simulink model "unicycle_sd_mpc"  (R2021b)
settings: Solver=FixedStepAuto  StartTime=0.0  StopTime=simTime  RelTol=1e-3
values from neighbouring files (symbols this model uses):
  delta = Ts    [ChainedForm_mr.m]    (also in ChainedForm_sr.m = 1; initMoh.m = 1)
  deltabar = delta/2    (= 0.5)    [initMoh.m]
  ref0 = [0 0]    [initMoh.m]
  thetareference = pi/4    (= 0.785398163397)    [initMoh.m]
  Ts = deltabar    (= 0.5)    [initMoh.m]
  v0 = 0.5    [initMoh.m]
  x0 = [x01;x02;x03]    [initMoh.m]
libraries: mpclib x3
settings Model: Creator=mebbaid  LastModifiedBy=mebbaid
settings SolverCC: AlgebraicLoopSolver=TrustRegion
settings DataIOCC: ReturnWorkspaceOutputs=off
settings DebuggingCC: SignalInfNanChecking=error  SignalRangeChecking=error  ParameterUnderflowMsg=error  UniqueDataStoreMsg=error  SFMachineParentedDataDiag=warning  UnderSpecifiedDimensionMsg=warning  ArithmeticOperatorsInVariantConditions=warning
settings SFSimCC: CustomCodeUndefinedFunction=UseInterfaceOnly

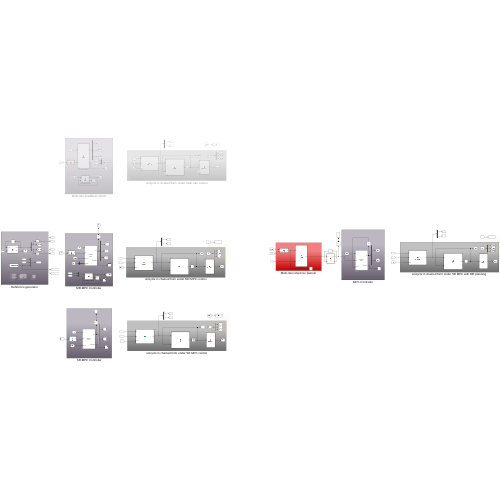
[thumbnail: Simulink's stored preview of the top-level diagram]
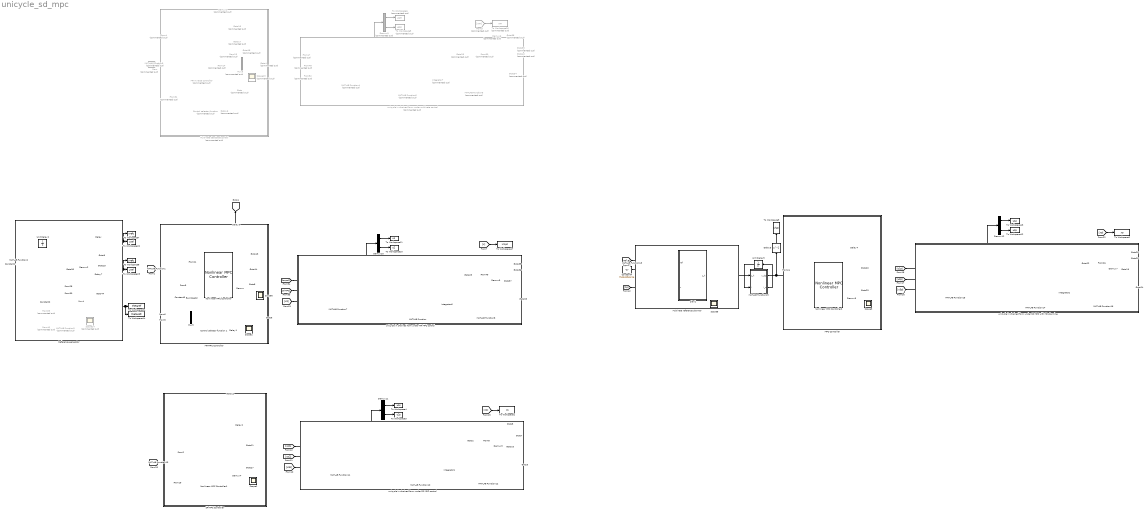
== system unicycle_sd_mpc ==
  Bus Creator : BusCreator  Inputs=1  OutDataTypeStr=Bus: myBusObject  NonVirtualBus=on
      settings: InheritFromInputs=off
  Constant1 : Constant  Value=v0
  Constant2 : Constant  Value=thetareference
  Constant3 : Constant  Value=Ts
  Constant4 : Constant  Value=thetareference
  "Control selector function " : MATLAB Function  Commented=on  TreatAsAtomicUnit=on  SystemSampleTime=deltabar
  Control selector function 1 : MATLAB Function  TreatAsAtomicUnit=on  SystemSampleTime=deltabar
  Delay : Delay  DelayLength=1  SampleTime=deltabar
  Delay1 : Delay  DelayLength=1  InitialCondition=1  SampleTime=deltabar
  Delay2 : Delay  DelayLength=1  InitialCondition=[0;0]  SampleTime=deltabar
  Delay3 : Delay  DelayLength=1  InitialCondition=[0;0;0]  SampleTime=delta
  Delay4 : Delay  DelayLength=1  InitialCondition=[0;0]  SampleTime=deltabar
  Delay5 : Delay  DelayLength=1  InitialCondition=[0 0 0]  SampleTime=delta
  Delay6 : Delay  Commented=on  DelayLength=1  InitialCondition=1  SampleTime=deltabar
  Delay7 : Delay  DelayLength=1  SampleTime=deltabar
  Demux{,3,5,7} (4 alike) : Demux  Outputs=3
  Demux1 : Demux  Commented=on  Outputs=3
  Demux{2,4,8,10..12} (6 alike) : Demux  Outputs=2
  Demux6 : Demux  Commented=on  Outputs=3
  Demux9 : Demux  Commented=on  Outputs=2
  From : From  Commented=on  GotoTag=refdes
  From13 : From  Commented=on  GotoTag=u21
  From14 : From  Commented=on  GotoTag=u22
  From3 : From  Commented=on  GotoTag=xm
  From31 : From  Commented=on  GotoTag=u2m
  From39 : From  Commented=on  GotoTag=xd
  From4 : From  Commented=on  GotoTag=zm
  From40 : From  Commented=on  GotoTag=yd
  From47 : From  Commented=on  GotoTag=u1
  From48 : From  Commented=on  GotoTag=u2_m
  From50 : From  Commented=on  GotoTag=xm
  From52 : From  Commented=on  GotoTag=x33
  Goto : Goto  Commented=on  GotoTag=u2_m
  Goto16 : Goto  Commented=on  GotoTag=u1
  Goto17 : Goto  Commented=on  GotoTag=u21
  Goto18 : Goto  Commented=on  GotoTag=u22
  Goto26 : Goto  Commented=on  GotoTag=xm
  Goto34 : Goto  Commented=on  GotoTag=zm
  Goto38 : Goto  Commented=on  GotoTag=x11
  Goto39 : Goto  Commented=on  GotoTag=x22
  Goto4 : Goto  Commented=on  GotoTag=u2m
  Goto40 : Goto  Commented=on  GotoTag=x33
  Integrator1 : Integrator  InitialCondition=x0
  Integrator2 : Integrator  InitialCondition=x0
  Integrator6 : Integrator  InitialCondition=x0
  Integrator7 : Integrator  Commented=on  InitialCondition=x0
  MATLAB Function : MATLAB Function  TreatAsAtomicUnit=on
  MATLAB Function1 : MATLAB Function  TreatAsAtomicUnit=on
  MATLAB Function10 : MATLAB Function  TreatAsAtomicUnit=on
  MATLAB Function11 : MATLAB Function  TreatAsAtomicUnit=on
  MATLAB Function12 : MATLAB Function  TreatAsAtomicUnit=on
  MATLAB Function13 : MATLAB Function  TreatAsAtomicUnit=on  SystemSampleTime=delta
  MATLAB Function14 : MATLAB Function  TreatAsAtomicUnit=on
  MATLAB Function15 : MATLAB Function  TreatAsAtomicUnit=on
  MATLAB Function16 : MATLAB Function  TreatAsAtomicUnit=on
  MATLAB Function18 : MATLAB Function  TreatAsAtomicUnit=on
  MATLAB Function19 : MATLAB Function  TreatAsAtomicUnit=on  SystemSampleTime=deltabar
  MATLAB Function2 : MATLAB Function  TreatAsAtomicUnit=on  SystemSampleTime=delta
  MATLAB Function3 : MATLAB Function  Commented=on  TreatAsAtomicUnit=on
  MATLAB Function4 : MATLAB Function  Commented=on  TreatAsAtomicUnit=on
  MATLAB Function5 : MATLAB Function  Commented=on  TreatAsAtomicUnit=on
  MATLAB Function6 : MATLAB Function  Commented=on  TreatAsAtomicUnit=on
  MATLAB Function7 : MATLAB Function  TreatAsAtomicUnit=on
  MATLAB Function8 : MATLAB Function  TreatAsAtomicUnit=on
  MATLAB Function9 : MATLAB Function  Commented=on  TreatAsAtomicUnit=on
  MPC Controller : Subsystem
  MR Inverse controller : MATLAB Function  Commented=on  TreatAsAtomicUnit=on  SystemSampleTime=delta
  MR-MPC Controller : Subsystem
  Multi-rate deadbeat control : Subsystem  Commented=on
  Multi-rate reference planner : Subsystem
  Mux3 : Mux  Commented=on  Inputs=2
  Mux4 : Mux  Inputs=3
  Mux5 : Mux  Inputs=2
  Nonlinear MPC Controller : mpclib/Nonlinear MPC Controller  SCDEnableBlockLinearizationSpecification=on  nlmpcobj=nlobj  UseObjectTs=on  TsControl=deltabar  UseMEX=off  md_enabled=off  mvtarget_enabled=off  param_enabled=on  cost_enabled=off  mvseq_enabled=off  stateseq_enabled=off  ovseq_enabled=off  slack_enabled=off  status_enabled=on  ov_min=off  ov_max=off  mv_min=off  mv_max=off  mvrate_min=off  mvrate_max=off  state_min=off  state_max=off  ov_weight=off  mv_weight=off  mvrate_weight=off  ecr_weight=off  nlp_initialize=off
  Nonlinear MPC Controller1 : mpclib/Nonlinear MPC Controller  SCDEnableBlockLinearizationSpecification=on  nlmpcobj=nlobjs  UseObjectTs=off  TsControl=deltabar  UseMEX=off  md_enabled=off  mvtarget_enabled=off  param_enabled=off  cost_enabled=off  mvseq_enabled=off  stateseq_enabled=off  ovseq_enabled=off  slack_enabled=off  status_enabled=on  ov_min=off  ov_max=off  mv_min=off  mv_max=off  mvrate_min=off  mvrate_max=off  state_min=off  state_max=off  ov_weight=off  mv_weight=off  mvrate_weight=off  ecr_weight=off  nlp_initialize=off
  Nonlinear MPC Controller2 : mpclib/Nonlinear MPC Controller  SCDEnableBlockLinearizationSpecification=on  nlmpcobj=nlobjp  UseObjectTs=on  TsControl=deltabar  UseMEX=off  md_enabled=off  mvtarget_enabled=off  param_enabled=off  cost_enabled=off  mvseq_enabled=off  stateseq_enabled=off  ovseq_enabled=off  slack_enabled=off  status_enabled=on  ov_min=off  ov_max=off  mv_min=off  mv_max=off  mvrate_min=off  mvrate_max=off  state_min=off  state_max=off  ov_weight=off  mv_weight=off  mvrate_weight=off  ecr_weight=off  nlp_initialize=off
  Reference generator : Subsystem
  SR-MPC Controller : Subsystem
  Scope{1..3,5..6} (5 alike) : Scope
  Scope13 : Scope  Commented=on
  Scope14 : Scope  Commented=on
  To Workspace1 : ToWorkspace  VariableName=xs  SampleTime=10^-3
      settings: Save2DSignal=2-D array (concatenate along first dimension)
  To Workspace10 : ToWorkspace  VariableName=u2  SampleTime=10^-3
      settings: Save2DSignal=2-D array (concatenate along first dimension)
  To Workspace11 : ToWorkspace  VariableName=u1  SampleTime=10^-3
      settings: Save2DSignal=2-D array (concatenate along first dimension)
  To Workspace12 : ToWorkspace  VariableName=u2p  SampleTime=10^-3
      settings: Save2DSignal=2-D array (concatenate along first dimension)
  To Workspace13 : ToWorkspace  VariableName=u1p  SampleTime=10^-3
      settings: Save2DSignal=2-D array (concatenate along first dimension)
  To Workspace14 : ToWorkspace  VariableName=thetarefc  SampleTime=10^-3
      settings: Save2DSignal=2-D array (concatenate along first dimension)
  To Workspace16 : ToWorkspace  Commented=on  VariableName=xm  SampleTime=10^-3
      settings: Save2DSignal=2-D array (concatenate along first dimension)
  To Workspace17 : ToWorkspace  VariableName=xmpc  SampleTime=10^-3
      settings: Save2DSignal=2-D array (concatenate along first dimension)
  To Workspace2 : ToWorkspace  VariableName=xp  SampleTime=10^-3
      settings: Save2DSignal=2-D array (concatenate along first dimension)
  To Workspace22 : ToWorkspace  VariableName=xref  SampleTime=delta
      settings: Save2DSignal=2-D array (concatenate along first dimension)
  To Workspace23 : ToWorkspace  VariableName=yref  SampleTime=delta
      settings: Save2DSignal=2-D array (concatenate along first dimension)
  To Workspace24 : ToWorkspace  VariableName=thetaref  SampleTime=delta
      settings: Save2DSignal=2-D array (concatenate along first dimension)
  To Workspace3 : ToWorkspace  VariableName=u2s  SampleTime=10^-3
      settings: Save2DSignal=2-D array (concatenate along first dimension)
  To Workspace4 : ToWorkspace  VariableName=u1s  SampleTime=10^-3
      settings: Save2DSignal=2-D array (concatenate along first dimension)
  To Workspace5 : ToWorkspace  Commented=on  VariableName=u2m  SampleTime=10^-3
      settings: Save2DSignal=2-D array (concatenate along first dimension)
  To Workspace6 : ToWorkspace  Commented=on  VariableName=u1m  SampleTime=10^-3
      settings: Save2DSignal=2-D array (concatenate along first dimension)
  To Workspace7 : ToWorkspace  VariableName=xrefc  SampleTime=10^-3
      settings: Save2DSignal=2-D array (concatenate along first dimension)
  To Workspace8 : ToWorkspace  VariableName=yrefc  SampleTime=10^-3
      settings: Save2DSignal=2-D array (concatenate along first dimension)
  To Workspace9 : ToWorkspace  VariableName=yhat  SampleTime=delta
      settings: Save2DSignal=2-D array (concatenate along first dimension)
  Unit Delay2 : UnitDelay  InitialCondition=ref0  SampleTime=deltabar*2  HasFrameUpgradeWarning=on
  Unit Delay5 : UnitDelay  InitialCondition=1  SampleTime=deltabar  HasFrameUpgradeWarning=on
  plan1 : MATLAB Function  TreatAsAtomicUnit=on  SystemSampleTime=delta
  unicycle in chained form under MR MPC control : Subsystem
  unicycle in chained form under SR MPC control : Subsystem
  "unicycle in chained form under SR MPC with MR planning " : Subsystem
  unicycle in chained form under multi-rate control : Subsystem  Commented=on
  wires:
  Nonlinear MPC Controller/1 -> Delay3/1, Demux/1
  Demux/1 -> [cmpc1]
  Demux/2 -> [cmpc2]
  Demux1/2 -> Goto17/1
  MR Inverse controller/1(ctrl) -> Demux1/1
  Demux1/3 -> Goto18/1
  Delay6/1 -> "Control selector function "/2(i)
  "Control selector function "/2(i_new) -> Delay6/1
  From31/1 -> "Control selector function "/1(u)
  Mux3/1 -> Goto4/1
  From13/1 -> Mux3/1
  From14/1 -> Mux3/2
  Demux/3 -> [cmpc3]
  "Control selector function "/1(y) -> Goto/1
  Demux1/1 -> Goto16/1
  Nonlinear MPC Controller/2 -> Scope6/1
  Unit Delay2/1 -> MATLAB Function2/1(ref_old)
  MATLAB Function2/2(ref_x) -> [ref_e]
  Constant1/1 -> MATLAB Function2/2(v0)
  Bus Creator/1 -> Nonlinear MPC Controller/4
  Constant3/1 -> Bus Creator/1
  From39/1 -> MATLAB Function3/1(xd)
  From40/1 -> MATLAB Function3/2(yd)
  MR Inverse controller/2(e) -> Scope13/1
  MATLAB Function3/1(thetad) -> Scope14/1
  MATLAB Function/1(xd) -> Integrator6/1
  MATLAB Function6/1(xd) -> Integrator7/1
  Integrator6/1 -> [x], MATLAB Function/2(x), MATLAB Function8/1(x)
  Integrator7/1 -> MATLAB Function5/1(x), Goto26/1, MATLAB Function6/2(x)
  MATLAB Function8/1(z) -> [z]
  MATLAB Function5/1(z) -> Goto34/1
  [x] -> Demux5/1
  Demux6/2 -> Goto39/1
  Demux5/3 -> [x3]
  Demux5/2 -> [x2]
  Demux6/1 -> Goto38/1
  From50/1 -> Demux6/1
  Demux6/3 -> Goto40/1
  Demux5/1 -> [x1]
  [x3] -> MATLAB Function7/3(theta)
  From52/1 -> MATLAB Function4/3(theta)
  MATLAB Function4/1(inp) -> Demux9/1, MATLAB Function6/1(u)
  MATLAB Function9/1(ref) -> MR Inverse controller/2(ref)
  MATLAB Function1/1(ref) -> Nonlinear MPC Controller/2
  [refdes] -> MATLAB Function1/1(xd)
  From47/1 -> MATLAB Function4/1(u1)
  From48/1 -> MATLAB Function4/2(u2)
  [ctrlMPC] -> MATLAB Function7/2(u2)
  [cmpc1] -> MATLAB Function7/1(u1)
  [z] -> Nonlinear MPC Controller/1
  Delay3/1 -> [umpc]
  [umpc] -> Nonlinear MPC Controller/3
  Control selector function 1/1(y) -> [ctrlMPC]
  Mux5/1 -> Control selector function 1/1(u)
  Control selector function 1/2(i_new) -> Delay1/1
  Delay1/1 -> Scope2/1, Control selector function 1/2(i)
  [cmpc3] -> Mux5/2
  [cmpc2] -> Mux5/1
  Demux2/1 -> Delay/1, [xd]
  Demux2/2 -> Delay7/1, [yd]
  MATLAB Function2/1(ref_x1) -> Demux2/1, Unit Delay2/1
  Delay7/1 -> To Workspace8/1, To Workspace23/1
  Delay/1 -> To Workspace7/1, To Workspace22/1
  Mux4/1 -> [refdes]
  [xd] -> Mux4/1
  [yd] -> Mux4/2
  From/1 -> MATLAB Function9/1(xd)
  From4/1 -> MR Inverse controller/1(xk)
  From3/1 -> To Workspace16/1
  [x] -> To Workspace17/1
  [xs] -> To Workspace1/1
  MATLAB Function10/1(xd) -> Integrator1/1
  [us1] -> MATLAB Function11/1(u1)
  [us2] -> MATLAB Function11/2(u2)
  Demux3/2 -> [x2s]
  [xs] -> Demux3/1
  Integrator1/1 -> [xs], MATLAB Function10/2(x), MATLAB Function12/1(x)
  MATLAB Function12/1(z) -> [zs]
  Demux3/1 -> [x1s]
  Demux3/3 -> [x3s]
  [x3s] -> MATLAB Function11/3(theta)
  MATLAB Function13/1(ref) -> Nonlinear MPC Controller1/2
  Nonlinear MPC Controller1/1 -> Demux4/1, Delay2/1
  Demux4/2 -> [us2]
  Nonlinear MPC Controller1/2 -> Scope1/1
  [refdes] -> MATLAB Function13/1(xd)
  Demux4/1 -> [us1]
  [zs] -> Nonlinear MPC Controller1/1
  Delay2/1 -> [us]
  [us] -> Nonlinear MPC Controller1/3
  [x3p] -> MATLAB Function15/3(theta)
  Demux7/1 -> [x1p]
  MATLAB Function16/1(z) -> [zp]
  [xp] -> Demux7/1
  Demux7/2 -> [x2p]
  Integrator2/1 -> [xp], MATLAB Function14/2(x), MATLAB Function16/1(x)
  [u2p] -> MATLAB Function15/2(u2)
  MATLAB Function14/1(xd) -> Integrator2/1
  [xp] -> To Workspace2/1
  [zp] -> Nonlinear MPC Controller2/1
  Delay4/1 -> Nonlinear MPC Controller2/3
  Demux7/3 -> [x3p]
  Demux8/2 -> [u2p]
  [u1p] -> MATLAB Function15/1(u1)
  Nonlinear MPC Controller2/1 -> Demux8/1, Delay4/1
  Demux8/1 -> [u1p]
  Nonlinear MPC Controller2/2 -> Scope3/1
  [ref_e] -> MATLAB Function18/1(ref_e)
  MATLAB Function18/1(ref) -> plan1/1(ref), Scope5/1
  [zp] -> plan1/2(x)
  Constant4/1 -> MATLAB Function18/2(theta_d)
  Unit Delay5/1 -> MATLAB Function19/2(i)
  MATLAB Function19/2(i_n) -> Unit Delay5/1
  plan1/1(z_h) -> MATLAB Function19/1(z_h)
  MATLAB Function19/1(x_dp) -> Nonlinear MPC Controller2/2, Delay5/1
  Delay5/1 -> To Workspace9/1
  Demux9/1 -> To Workspace6/1
  Demux9/2 -> To Workspace5/1
  MATLAB Function7/1(inp) -> Demux10/1, MATLAB Function/1(u)
  Demux10/2 -> To Workspace10/1
  Demux10/1 -> To Workspace11/1
  MATLAB Function11/1(inp) -> Demux11/1, MATLAB Function10/1(u)
  Demux11/2 -> To Workspace3/1
  Demux11/1 -> To Workspace4/1
  MATLAB Function15/1(inp) -> Demux12/1, MATLAB Function14/1(u)
  Demux12/2 -> To Workspace12/1
  Demux12/1 -> To Workspace13/1
  Constant2/1 -> Mux4/3, To Workspace14/1, To Workspace24/1

== system unicycle_sd_mpc/MPC Controller ==

== system unicycle_sd_mpc/MR-MPC Controller ==

== system unicycle_sd_mpc/Multi-rate deadbeat control ==

== system unicycle_sd_mpc/Multi-rate reference planner ==

== system unicycle_sd_mpc/Reference generator ==

== system unicycle_sd_mpc/SR-MPC Controller ==

== system unicycle_sd_mpc/unicycle in chained form under MR MPC control ==

== system unicycle_sd_mpc/unicycle in chained form under SR MPC control ==

== system unicycle_sd_mpc/unicycle in chained form under SR MPC with MR planning  ==

== system unicycle_sd_mpc/unicycle in chained form under multi-rate control ==

== matlab function unicycle_sd_mpc/MATLAB Function7 ==
  data: u1 input; inp output; u2 input; theta input; scneario parameter
function inp = InTxAct1(u1,u2, theta, scneario)
if scneario == 1
    v = u1/cos(theta);
    w = u2*(cos(theta))^2;
else
    v = u1;
    w = u2;
end
    inp = [v;w];
%%

== matlab function unicycle_sd_mpc/MATLAB Function8 ==
  data: x input; z output
function z = StatesTx1(x)
%% Define the input Tx here
z = zeros(3,1);
z(1) = x(1);
z(2) = tan(x(3));
z(3) = x(2);

== matlab function unicycle_sd_mpc/MATLAB Function9 ==
  data: xd input; ref output
function ref = refTx(xd)

ref = [xd(1);tan(xd(3));xd(2)];

== matlab function unicycle_sd_mpc/MATLAB Function10 ==
  data: u input; xd output; x input
function xd = Dyn1(u,x)
xd = zeros(3,1);
inp = u;
xd(1) = cos(x(3))*inp(1);
xd(2) = sin(x(3))*inp(1);
xd(3) = inp(2);

== matlab function unicycle_sd_mpc/MATLAB Function11 ==
  data: u1 input; inp output; u2 input; theta input; scneario parameter
function inp = InTxAct1(u1,u2, theta, scneario)
if scneario == 1
    v = u1/cos(theta);
    w = u2*(cos(theta))^2;
else
    v = u1;
    w = u2;
end
    inp = [v;w];
%% 

%%

== matlab function unicycle_sd_mpc/MATLAB Function5 ==
  data: x input; z output
function z = StatesTx2(x)
%% Define the input Tx here
z = zeros(3,1);
z(1) = x(1);
z(2) = tan(x(3));
z(3) = x(2);

== matlab function unicycle_sd_mpc/MATLAB Function12 ==
  data: x input; z output
function z = StatesTx1(x)
%% Define the input Tx here
z = zeros(3,1);
z(1) = x(1);
z(2) = tan(x(3));
z(3) = x(2);

== matlab function unicycle_sd_mpc/MATLAB Function13 ==
  data: ref output; xd input; thetareference parameter
function ref = fcn(xd, thetareference)
ref = [xd(1) tan(xd(3)) xd(2)];

== matlab function unicycle_sd_mpc/MATLAB Function15 ==
  data: u1 input; inp output; u2 input; theta input; scneario parameter
function inp = InTxAct1(u1,u2, theta, scneario)
%inp = u;

if scneario == 1
    v = u1/cos(theta);
    w = u2*(cos(theta))^2;
else
    v = u1;
    w = u2;
end
    inp = [v;w];

%%

== matlab function unicycle_sd_mpc/MATLAB Function16 ==
  data: x input; z output
function z = StatesTx1(x)
%% Define the input Tx here
z = zeros(3,1);
z(1) = x(1);
z(2) = tan(x(3));
z(3) = x(2);

== matlab function unicycle_sd_mpc/MATLAB Function18 ==
  data: ref_e input; ref output; theta_d input
function ref = refTx(ref_e, theta_d)


ref = [ref_e(1,:);tan(theta_d) tan(theta_d); ref_e(2,:)];

== matlab function unicycle_sd_mpc/MATLAB Function19 ==
  data: x_dp output; z_h input; i_n output; i input
function [x_dp,i_n] = fcn(z_h, i)


if i <2
    i_n = i+1; 
else 
    i_n = 1; 
end
%

aux = z_h(:, i:i+1);
z_d = transpose(aux);

x_d = zeros(2,3);
xx = z_d(1,:);
x_dp = z_d(1,:);

== matlab function unicycle_sd_mpc/MATLAB Function4 ==
  data: u1 input; inp output; u2 input; theta input; scneario parameter
function inp = InTxAct2(u1,u2, theta, scneario)
%inp = u;
if scneario == 1
    v = u1/cos(theta);
    w = u2*(cos(theta))^2;
else
    v = u1;
    w = u2;
end
    inp = [v;w];

%%

== matlab function unicycle_sd_mpc/plan1 ==
  data: z_h output; ref input; deltabar parameter; x input; delta parameter

function z_h =  plan1(ref, deltabar, x, delta)

z_h  = zeros(3,4);
ref1 = ref(:,1);
ref2 = ref(:,2); 
z_t  = x; 


% First step
u11 = (ref1(1)-x(1))/delta;

Ad = [1 0;deltabar*u11 1];
bd =  [deltabar;((deltabar^2)/2)*u11];
A1 = Ad^2;
B1 = [Ad*bd bd];

u12 = inv(B1)*(ref1(2:3)-A1*x(2:3));
u1  = [u11;u12];

u_1 = [u11 u11;u12']; 

% Second step

x1 = x(1) + 2*deltabar*u11;
x2 = x(2) +  deltabar*(u12(1)+ u12(2));
x3 = x(3) +  2*deltabar*x(2)*u11 + 3*deltabar^2/2*u11*u12(1)+deltabar^2/2*u11*u12(2);

u21 = (ref2(1)-x1(1))/delta;
u22 = inv(B1)*(ref2(2:3)-A1*[x2;x3]);  
u2  = [u21;u22];

u_2 = [u21 u21;u22']; 

u_p = [u_1  u_2];




% Applying uhat
% First iteration
 z     = z_t;  
 
 ztmp1 = z(1) + deltabar*u_p(1,1);
 ztmp2 = z(2) + deltabar*u_p(2,1);
 ztmp3 = z(3) + deltabar*u_p(1,1)*z(2)+deltabar^2/2*u_p(1,1)*u_p(2,1);
 
 z_h(:,1) = [ztmp1;ztmp2;ztmp3]; 
 
 for i = 2:4
     A = [1 0;deltabar*u_p(1,i) 1];
     B = [deltabar;((deltabar^2)/2)*u_p(1,i)];
     z_h(1,i)   = z_h(1,i-1) + deltabar*u_p(1,i);
     z_h(2:3,i) = A*z_h(2:3,i-1) + B*u_p(2,i);
 end
end

== matlab function unicycle_sd_mpc/MR Inverse controller ==
  data: xk input; ctrl output; ref input; delta parameter; e output

function [ctrl ,e] =  control(xk,ref,delta)
%delta = 1;
deltabar = delta/2;

u1 = (ref(1)-xk(1))/delta;
A = [1 0;deltabar*u1 1];
B = [deltabar;((deltabar^2)/2)*u1];
R = [A*B B];
e = [ref(2);ref(3)]-A^2*[xk(2);xk(3)];
u = pinv(R)*e;
ctrl = [u1;u];

end

== matlab function unicycle_sd_mpc/Control selector function 1 ==
  data: u input; y output; i input; i_new output
function [y, i_new] = fcn(u, i)

if i< 2
i_new = i+1;
else
i_new = 1;
end
y = u(i);

== matlab function unicycle_sd_mpc/MATLAB Function2 ==
  data: ref_x1 output; ref_old input; ref_x output size=[2;2]; v0 input; deltabar parameter
function [ref_x1,ref_x] = fcn(ref_old, v0, deltabar)
delta = deltabar*2; 
a1 = 1;
a2 = 1;

%ref1 = ref_old+delta*v0*[a1; a1 a2];
% ref_old(2) = 0; 
% ref_old(4) = 0; 
% ref_old(5:6) = [0; 0];

ref_x1 = ref_old + [delta*v0*a1;delta*v0*a2];

ref_x2 = ref_x1 + [delta*v0*a1;delta*v0*a2];

ref_x = [ref_x1 ref_x2];

== matlab function unicycle_sd_mpc/Control selector function  ==
  data: u input; y output; i input; i_new output
function [y, i_new] = fcn(u, i)

if i< 2
i_new = i+1;
else
i_new = 1;
end
y = u(i);

== matlab function unicycle_sd_mpc/MATLAB Function14 ==
  data: u input; xd output; x input
function xd = Dyn1(u,x)
xd = zeros(3,1);
inp = u;
xd(1) = cos(x(3))*inp(1);
xd(2) = sin(x(3))*inp(1);
xd(3) = inp(2);

== matlab function unicycle_sd_mpc/MATLAB Function ==
  data: u input; xd output; x input
function xd = Dyn1(u,x)
xd = zeros(3,1);
inp = u;
xd(1) = cos(x(3))*inp(1);
xd(2) = sin(x(3))*inp(1);
xd(3) = inp(2);

== matlab function unicycle_sd_mpc/MATLAB Function3 ==
  data: xd input; thetad output; yd input
function thetad = fcn(xd,yd)

thetad = atan2(yd,xd);

== matlab function unicycle_sd_mpc/MATLAB Function1 ==
  data: xd input; ref output
function ref = refTxmPC(xd)

ref = [xd(1) tan(xd(3)) xd(2)];

== matlab function unicycle_sd_mpc/MATLAB Function6 ==
  data: u input; xd output; x input
function xd = Dyn2(u,x)
xd = zeros(3,1);
inp = u;


%% 
xd(1) = cos(x(3))*inp(1);
xd(2) = sin(x(3))*inp(1);
xd(3) = inp(2);
